simulink model "JX_Kinect20131119"  (Simulink 7.7)
settings: Solver=ode4  StartTime=0.0  StopTime=inf  FixedStep=sample_time  RelTol=1e-3
InitFcn:
  | sample_time=0.005;%0.004;%0.0025;%0.02;
  | DeltaT = 0.02;
  | g = 9.81;
  | H0 = g%0.3165;
  | Kl = 1;
  | 
  | Omega_r = 1.6;%for Horizontal reference
  | Zeta_r = 1; %for Horizontal reference
  | Omega = 1.8;%for Horizontal Control
  | Zeta = 0.5;    %for Horizontal Control
  | 
  | Omega_h_r = 2.5; %for vertical reference
  | Zeta_h_r = 0.8;  %for vertical reference
  | Omega_h = 2.7;    %for vertical control
  | Zeta_h = 0.8;         %for vertical control
  | PI=pi;
  | 
  | Mass = 1.15;
  | Acc_Max = 4;
  | Acc_Max_h = 4;
  | 
  | Max_RP = 60;
  | 
  | % for NN
  | n = 5;
  | r = 3;
  | n2 = 5;
  | NN_ST = 0.02;
  | 
  | GAMA_V = 6;
  | gama_V_e = 0.01;
  | 
  | GAMA_W = GAMA_V;
  | gama_W_e =0.01;
  | 
  | % deadzone
  | NN_Deadzone_Z = 0;
  | 
  | % inputs nomalizaton parameters
  | NN_Z_y_min = -3;
  | NN_Z_y_max = 0.5;
  | 
  | NN_Z_v_max = 8;
  | NN_Z_v_min = -NN_Z_v_max;
  | 
  | % alpha = 0.034;
  | alpha = 1;
  | % c_f = 0.0015;
  | c_f = 0.001;
  | c_y_tilt = 1*0.5;
  | 
  | %for WK paras
  | Heightcontrol = 0.08;
  | Scale_Factor=1;
  | yoffset=0;
  | 
  | load MaoBi_Oct04_2_int.mat
  | MB_Interp.time = [];
undefined symbols (not defined in the file or in its folder): DiscIntNeverNeededParam
libraries: simulink x7, dspadpt3 x3, nid_lib x2, X330_Control x2
(part 2 of 2)

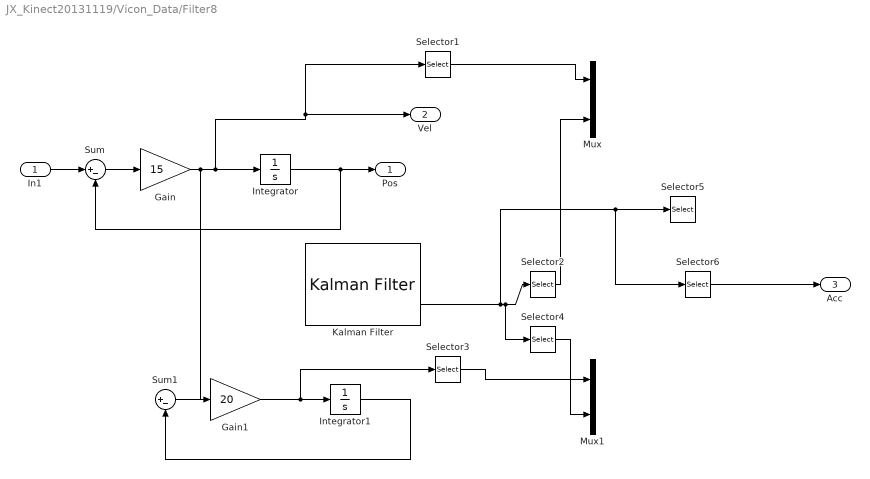
== system JX_Kinect20131119/Vicon_Data/Filter8 ==
  In1 : Inport
  Gain : Gain  Gain=15
  Gain1 : Gain  Gain=20
  Integrator : Integrator
  Integrator1 : Integrator
  Kalman Filter : dspadpt3/Kalman Filter  SystemSampleTime=-1  num_targets=1  sourceEnable=Always  isReset=on  X=zeros([9, 1])  P=zeros(9)  A=[1 sample_time sample_time*sample_time/2 zeros(1,6);0 1 sample_time zeros(1,6);0 0 1 zeros(1,6);0 0 0 1 sample_time sample_time*sample_time/2 0 0 0;zeros(1,4) 1 sample_time zeros(1,3);zeros(1,5) 1 zeros(1,3);zeros(1,6) 1 sample_time sample_time*sample_time/2;zeros(1,7) 1 sample_time;zeros(1,8) 1]  sourceMeasure=Specify via Dialog  H=[1 zeros(1,8); zeros(1,3) 1 zeros(1,5);zeros(1,6) 1 0 0]  Q=diag([0 0.001 0.001 0 0.001 0.001 0 0.001 0.001])  R=0.001*eye(3)  isOutputEstMeasure=on  isOutputEstState=on  isOutputEstError=off  isOutputPrdMeasure=off  isOutputPrdState=off  isOutputPrdError=off
  Mux : Mux  Inputs=2
  Mux1 : Mux  Inputs=2
  Selector1 : Selector  InputPortWidth=3  IndexOptions=Index vector (dialog)  Indices=[2]  OutputSizes=1
  Selector2 : Selector  InputPortWidth=9  IndexOptions=Index vector (dialog)  Indices=[5]  OutputSizes=1
  Selector3 : Selector  InputPortWidth=3  IndexOptions=Index vector (dialog)  Indices=[2]  OutputSizes=1
  Selector4 : Selector  InputPortWidth=9  IndexOptions=Index vector (dialog)  Indices=[6]  OutputSizes=1
  Selector5 : Selector  InputPortWidth=9  IndexOptions=Index vector (dialog)  Indices=[2 5 8]  OutputSizes=1
  Selector6 : Selector  InputPortWidth=9  IndexOptions=Index vector (dialog)  Indices=[3 6 9]  OutputSizes=1
  Sum : Sum  Inputs=|+-
  Sum1 : Sum  Inputs=|+-
  Pos : Outport
  Vel : Outport  Port=2
  Acc : Outport  Port=3
  wires:
  Selector6/1 -> Acc/1
  Selector4/1 -> Mux1/2
  Selector3/1 -> Mux1/1
  Selector2/1 -> Mux/2
  Integrator1/1 -> Sum1/2
  Gain1/1 -> Selector3/1, Integrator1/1
  Sum1/1 -> Gain1/1
  Kalman Filter/2 -> Selector6/1, Selector5/1, Selector2/1, Selector4/1
  Selector1/1 -> Mux/1
  In1/1 -> Sum/1
  Integrator/1 -> Sum/2, Pos/1
  Gain/1 -> Sum1/1, Vel/1, Selector1/1, Integrator/1
  Sum/1 -> Gain/1

== system JX_Kinect20131119/Vicon_Data/Raw Quad Pose from Vicon ==
  Constant : Constant
  Demux : Demux  Outputs=3
  Interpreted MATLAB Function : MATLABFcn  MATLABFcn=JXKinect05112013
  Process Vicon Raw Data1 : Subsystem
  Process Vicon Raw Data6 : Subsystem
  Process Vicon Raw Data7 : Subsystem
  Position_Vicon_JianXing : Outport
  Attitude_Vicon_JianXing : Outport  Port=2
  Position_Vicon_K platform : Outport  Port=3
  Attitude_Vicon_K platform : Outport  Port=4
  Position_Vicon_draw : Outport  Port=5
  Attitude_Vicon_draw : Outport  Port=6
  wires:
  Demux/3 -> Process Vicon Raw Data1/1(Vicon Raw)
  Process Vicon Raw Data1/1(Position) -> Position_Vicon_draw/1
  Process Vicon Raw Data1/2(Attitude) -> Attitude_Vicon_draw/1
  Demux/2 -> Process Vicon Raw Data7/1(Vicon Raw)
  Process Vicon Raw Data7/1(Position) -> Position_Vicon_K platform/1
  Process Vicon Raw Data7/2(Attitude) -> Attitude_Vicon_K platform/1
  Constant/1 -> Interpreted MATLAB Function/1
  Demux/1 -> Process Vicon Raw Data6/1(Vicon Raw)
  Process Vicon Raw Data6/1(Position) -> Position_Vicon_JianXing/1
  Process Vicon Raw Data6/2(Attitude) -> Attitude_Vicon_JianXing/1
  Interpreted MATLAB Function/1 -> Demux/1

== system JX_Kinect20131119/Kinect/Subsystem/Front or Center or Back ==
  Z: LH : Inport
  Z: LSh : Inport  Port=2
  Constant1 : Constant  Value=0
  Constant2 : Constant
  Constant3 : Constant  Value=-1
  If Back : Subsystem  TreatAsAtomicUnit=on
  If Center : Subsystem  TreatAsAtomicUnit=on
  If Front or Center or Back : If  IfExpression=u1 > 0.40  ElseIfExpressions=u1 >= 0.23
  If front : Subsystem  TreatAsAtomicUnit=on
  Merge3 : Merge  Inputs=3
  Subtract : Sum  Inputs=-+
  Y FrontCenterBack : Outport
  wires:
  Z: LH/1 -> Subtract/1
  Z: LSh/1 -> Subtract/2
  If Front or Center or Back/1 -> If front/Action
  If Front or Center or Back/2 -> If Center/Action
  If Front or Center or Back/3 -> If Back/Action
  If front/1(Out1) -> Merge3/1
  If Center/1(Out1) -> Merge3/2
  Constant2/1 -> If front/1(In1)
  Constant1/1 -> If Center/1(In1)
  Constant3/1 -> If Back/1(In1)
  If Back/1(Out1) -> Merge3/3
  Merge3/1 -> Y FrontCenterBack/1
  Subtract/1 -> If Front or Center or Back/1

== system JX_Kinect20131119/Kinect/Subsystem/Left or Center or Right ==
  X: LH : Inport
  X: LSh : Inport  Port=2
  Dead Zone : DeadZone  LowerValue=-0.14  UpperValue=0.14  SaturateOnIntegerOverflow=on
  Gain : Gain  Gain=2000
  Saturation : Saturate  UpperLimit=1  LowerLimit=-1
  Subtract : Sum  Inputs=+-
  X LeftCenterRight : Outport
  wires:
  X: LSh/1 -> Subtract/2
  X: LH/1 -> Subtract/1
  Subtract/1 -> Dead Zone/1
  Dead Zone/1 -> Gain/1
  Gain/1 -> Saturation/1
  Saturation/1 -> X LeftCenterRight/1

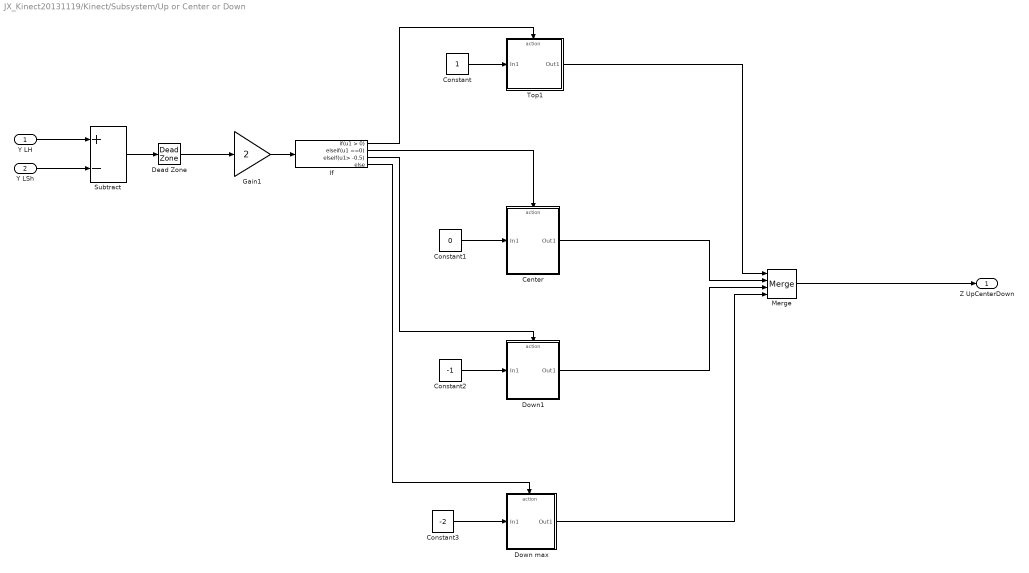
== system JX_Kinect20131119/Kinect/Subsystem/Up or Center or Down ==
  Y LH : Inport
  Y LSh : Inport  Port=2
  Center : Subsystem  TreatAsAtomicUnit=on
  Constant : Constant
  Constant1 : Constant  Value=0
  Constant2 : Constant  Value=-1
  Constant3 : Constant  Value=-2
  Dead Zone : DeadZone  LowerValue=-0.12  UpperValue=0.12  SaturateOnIntegerOverflow=on
  Down max : Subsystem  TreatAsAtomicUnit=on
  Down1 : Subsystem  TreatAsAtomicUnit=on
  Gain1 : Gain  Gain=2
  If : If  ElseIfExpressions=u1 ==0, u1> -0.5
  Merge : Merge  Inputs=4
  Subtract : Sum  Inputs=+-
  Top1 : Subsystem  TreatAsAtomicUnit=on
  Z UpCenterDown : Outport
  wires:
  Subtract/1 -> Dead Zone/1
  If/1 -> Top1/Action
  If/2 -> Center/Action
  If/3 -> Down1/Action
  If/4 -> Down max/Action
  Constant/1 -> Top1/1(In1)
  Dead Zone/1 -> Gain1/1
  Gain1/1 -> If/1
  Constant1/1 -> Center/1(In1)
  Constant2/1 -> Down1/1(In1)
  Constant3/1 -> Down max/1(In1)
  Center/1(Out1) -> Merge/2
  Down1/1(Out1) -> Merge/3
  Down max/1(Out1) -> Merge/4
  Top1/1(Out1) -> Merge/1
  Merge/1 -> Z UpCenterDown/1
  Y LH/1 -> Subtract/1
  Y LSh/1 -> Subtract/2

== system JX_Kinect20131119/Kinect/Subsystem1/Left or Center or Right ==
  X: RH : Inport
  X: RSh : Inport  Port=2
  Dead Zone : DeadZone  LowerValue=-0.12  UpperValue=0.12  SaturateOnIntegerOverflow=on
  Gain : Gain  Gain=2000
  Saturation : Saturate  UpperLimit=1  LowerLimit=-1
  Subtract : Sum  Inputs=+-
  LeftCenterRight : Outport
  wires:
  X: RSh/1 -> Subtract/2
  Subtract/1 -> Dead Zone/1
  Dead Zone/1 -> Gain/1
  Gain/1 -> Saturation/1
  Saturation/1 -> LeftCenterRight/1
  X: RH/1 -> Subtract/1

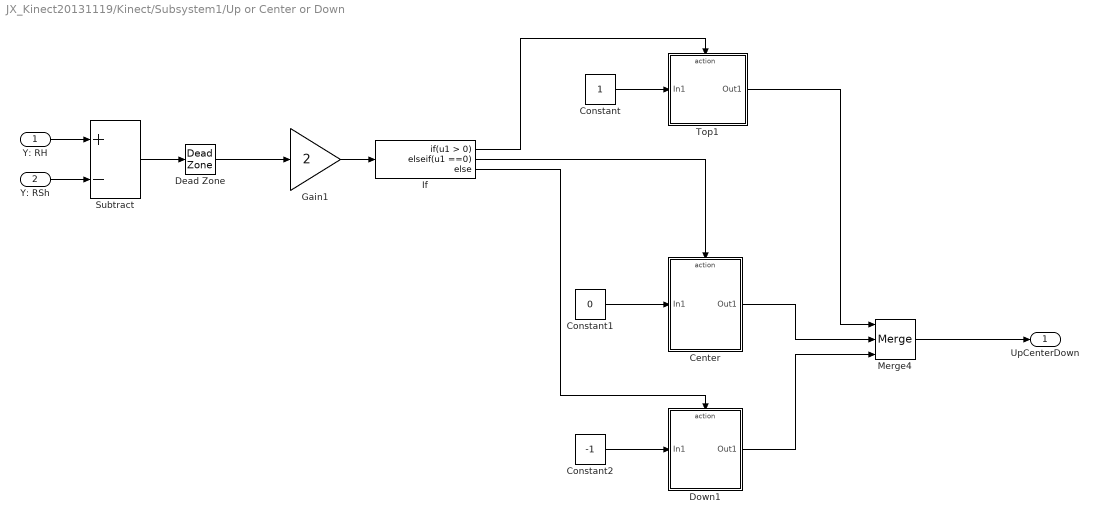
== system JX_Kinect20131119/Kinect/Subsystem1/Up or Center or Down ==
  Y: RH : Inport
  Y: RSh : Inport  Port=2
  Center : Subsystem  TreatAsAtomicUnit=on
  Constant : Constant
  Constant1 : Constant  Value=0
  Constant2 : Constant  Value=-1
  Dead Zone : DeadZone  LowerValue=-0.12  UpperValue=0.12  SaturateOnIntegerOverflow=on
  Down1 : Subsystem  TreatAsAtomicUnit=on
  Gain1 : Gain  Gain=2
  If : If  ElseIfExpressions=u1 ==0
  Merge4 : Merge  Inputs=3
  Subtract : Sum  Inputs=+-
  Top1 : Subsystem  TreatAsAtomicUnit=on
  UpCenterDown : Outport
  wires:
  Subtract/1 -> Dead Zone/1
  If/1 -> Top1/Action
  If/2 -> Center/Action
  Constant/1 -> Top1/1(In1)
  Dead Zone/1 -> Gain1/1
  Gain1/1 -> If/1
  Constant1/1 -> Center/1(In1)
  Constant2/1 -> Down1/1(In1)
  Center/1(Out1) -> Merge4/2
  Down1/1(Out1) -> Merge4/3
  Top1/1(Out1) -> Merge4/1
  Merge4/1 -> UpCenterDown/1
  Y: RH/1 -> Subtract/1
  Y: RSh/1 -> Subtract/2
  If/3 -> Down1/Action

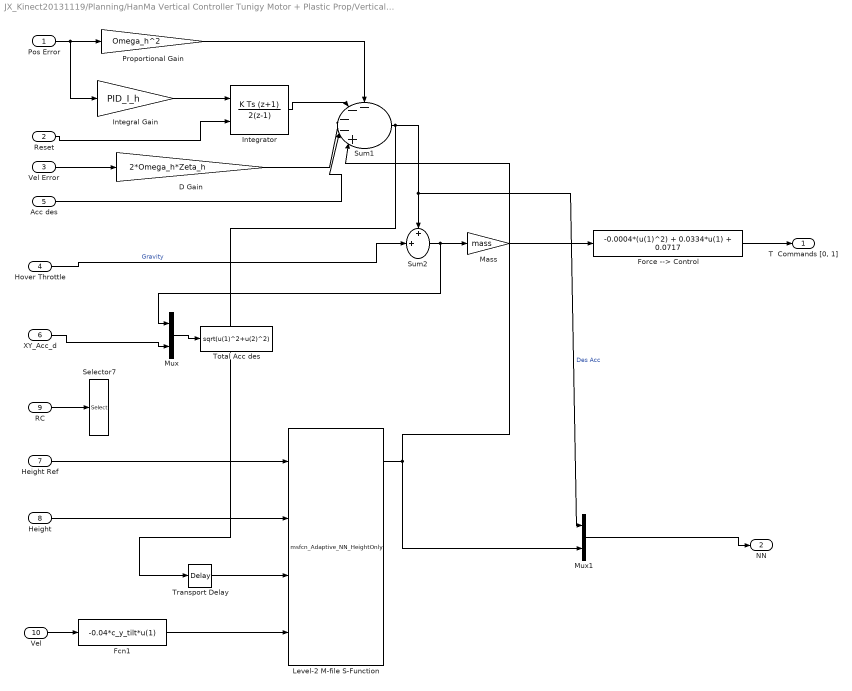
== system JX_Kinect20131119/Planning/HanMa Vertical Controller Tunigy Motor + Plastic Prop/Verticall Pos Controller ==
  Pos Error : Inport
  Reset : Inport  Port=2
  Vel Error : Inport  Port=3
  Hover Throttle : Inport  Port=4
  Acc des : Inport  Port=5
  XY_Acc_d : Inport  Port=6
  Height Ref : Inport  Port=7
  Height : Inport  Port=8
  RC : Inport  Port=9
  Vel : Inport  Port=10
  D Gain : Gain  Gain=2*Omega_h*Zeta_h  OutDataTypeStr=double
  Fcn1 : Fcn  Expr=-0.04*c_y_tilt*u(1)
  Force --> Control : Fcn  Expr=-0.0004*(u(1)^2) + 0.0334*u(1) + 0.0717
  Integral Gain : Gain  DisableCoverage=on  Gain=PID_I_h  ParamDataTypeStr=double  OutDataTypeStr=double
  Integrator : DiscreteIntegrator  DisableCoverage=on  IntegratorMethod=Integration: Trapezoidal  ExternalReset=rising  InitialConditionMode=State only (most efficient)  SampleTime=-1  OutDataTypeStr=double  UpperSaturationLimit=0.3  LowerSaturationLimit=-0.3  ICPrevOutput=DiscIntNeverNeededParam  ICPrevScaledInput=DiscIntNeverNeededParam
  Level-2 M-file S-Function : M-S-Function  FunctionName=msfcn_Adaptive_NN_HeightOnly  Parameters=n,r,n2,NN_ST,GAMA_V,gama_V_e,GAMA_W,gama_W_e,alpha,c_f,c_y_tilt,NN_Deadzone_Z,NN_Z_y_min,NN_Z_y_max,NN_Z_v_min,NN_Z_v_max
      mask Display: fprintf('Output Feedback NN \n Control Block')
  Mass : Gain  DisableCoverage=on  Gain=mass  ParamDataTypeStr=double  OutDataTypeStr=double
  Mux : Mux  Inputs=2
  Mux1 : Mux  Inputs=2
  Proportional Gain : Gain  DisableCoverage=on  Gain=Omega_h^2  ParamDataTypeStr=double  OutDataTypeStr=double
  Selector7 : Selector  InputPortWidth=8  IndexOptions=Index vector (dialog)  Indices=[6]  OutputSizes=1
  Sum1 : Sum  DisableCoverage=on  Inputs=----+|  AccumDataTypeStr=double  OutDataTypeStr=double  SampleTime=0.02
  Sum2 : Sum  DisableCoverage=on  Inputs=++|  AccumDataTypeStr=double  OutDataTypeStr=double  SampleTime=0.02
  Total Acc des : Fcn  Expr=sqrt(u(1)^2+u(2)^2)
  Transport Delay : TransportDelay  DelayTime=0.02
  "T  Commands [0, 1]" : Outport
  NN : Outport  Port=2
  wires:
  Force --> Control/1 -> "T  Commands [0, 1]"/1
  Sum2/1 -> Mux/1, Mass/1
  XY_Acc_d/1 -> Mux/2
  Mux/1 -> Total Acc des/1
  Mass/1 -> Force --> Control/1
  Sum1/1 -> Transport Delay/1, Sum2/1, Mux1/1  "Des Acc"
  Hover Throttle/1 -> Sum2/2  "Gravity"
  Acc des/1 -> Sum1/4
  D Gain/1 -> Sum1/3
  Vel Error/1 -> D Gain/1
  Reset/1 -> Integrator/2
  Pos Error/1 -> Integral Gain/1, Proportional Gain/1
  Proportional Gain/1 -> Sum1/1
  Integrator/1 -> Sum1/2
  Integral Gain/1 -> Integrator/1
  Height Ref/1 -> Level-2 M-file S-Function/1
  Level-2 M-file S-Function/1 -> Mux1/2, Sum1/5
  RC/1 -> Selector7/1
  Fcn1/1 -> Level-2 M-file S-Function/4
  Transport Delay/1 -> Level-2 M-file S-Function/3
  Mux1/1 -> NN/1
  Vel/1 -> Fcn1/1
  Height/1 -> Level-2 M-file S-Function/2

== system JX_Kinect20131119/Planning/Yaw Controller/Heading ==
  u : Inport  SampleTime=SampleTime
  RESET : Inport  Port=2  SampleTime=SampleTime
  Integral Gain : Gain  DisableCoverage=on  Gain=I  ParamMin=IParamMin  ParamMax=IParamMax  ParamDataTypeStr=IParamDataTypeStr  OutMin=IOutMin  OutMax=IOutMax  OutDataTypeStr=IOutDataTypeStr
  Integrator : DiscreteIntegrator  DisableCoverage=on  IntegratorMethod=Integration: Trapezoidal  ExternalReset=rising  InitialCondition=InitialConditionForIntegrator  InitialConditionMode=State only (most efficient)  SampleTime=-1  OutMin=IntegratorOutMin  OutMax=IntegratorOutMax  OutDataTypeStr=IntegratorOutDataTypeStr  ICPrevOutput=DiscIntNeverNeededParam  ICPrevScaledInput=DiscIntNeverNeededParam
  Proportional Gain : Gain  DisableCoverage=on  Gain=P  ParamMin=PParamMin  ParamMax=PParamMax  ParamDataTypeStr=PParamDataTypeStr  OutMin=POutMin  OutMax=POutMax  OutDataTypeStr=POutDataTypeStr
  Saturation : Saturate  UpperLimit=UpperSaturationLimit  LowerLimit=LowerSaturationLimit  LinearizeAsGain=off  OutMin=SaturationOutMin  OutMax=SaturationOutMax  OutDataTypeStr=SaturationOutDataTypeStr
  Sum : Sum  DisableCoverage=on  Inputs=++|  AccumDataTypeStr=SumAccumDataTypeStr  OutMin=SumOutMin  OutMax=SumOutMax  OutDataTypeStr=SumOutDataTypeStr
  y : Outport  InitialOutput=0
  wires:
  Sum/1 -> Saturation/1
  Saturation/1 -> y/1
  RESET/1 -> Integrator/2
  Proportional Gain/1 -> Sum/1
  Integrator/1 -> Sum/2
  Integral Gain/1 -> Integrator/1
  u/1 -> Proportional Gain/1, Integral Gain/1

== system JX_Kinect20131119/Vicon_Data/Raw Quad Pose from Vicon/Process Vicon Raw Data1 ==
  note: Z
  note: Y
  note: X
  Vicon Raw : Inport
  Add1 : Sum  Inputs=-+
  Constant1 : Constant  Value=pi  OutDataTypeStr=double
  Demux : Demux  Outputs=6
  Flip_pi1 : Subsystem
      mask Type: Flip -pi to pi
      mask Description: Flips the inputs into the range -pi to pi
      mask Help: Flips the inputs into the range -pi to pi
      mask Display: disp('Flip_pi')
  Gain1 : Gain  Gain=0.001
  Gain3 : Gain  Gain=-1
  Gain6 : Gain  Gain=-0.001
  Gain7 : Gain  Gain=-0.001
  Matrix Concatenate1 : Concatenate  NumInputs=3  Mode=Multidimensional array
  Matrix Concatenate13 : Concatenate  NumInputs=3  Mode=Multidimensional array
  Position : Outport
  Attitude : Outport  Port=2
  wires:
  Matrix Concatenate1/1 -> Attitude/1
  Vicon Raw/1 -> Demux/1
  Matrix Concatenate13/1 -> Position/1
  Flip_pi1/1(Angle_Flip) -> Matrix Concatenate1/1
  Demux/5 -> Matrix Concatenate1/2  "pitch"
  Gain3/1 -> Flip_pi1/1(Angle)
  Add1/1 -> Gain3/1
  Gain7/1 -> Matrix Concatenate13/3
  Gain6/1 -> Matrix Concatenate13/2
  Demux/4 -> Add1/1  "roll"
  Demux/3 -> Gain7/1
  Demux/2 -> Gain6/1
  Demux/1 -> Gain1/1
  Gain1/1 -> Matrix Concatenate13/1
  Demux/6 -> Matrix Concatenate1/3  "yaw"
  Constant1/1 -> Add1/2

== system JX_Kinect20131119/Vicon_Data/Raw Quad Pose from Vicon/Process Vicon Raw Data6 ==
  note: Z
  note: Y
  note: X
  Vicon Raw : Inport
  Add1 : Sum  Inputs=-+
  Constant1 : Constant  Value=pi  OutDataTypeStr=double
  Demux : Demux  Outputs=6
  Flip_pi1 : Subsystem
      mask Type: Flip -pi to pi
      mask Description: Flips the inputs into the range -pi to pi
      mask Help: Flips the inputs into the range -pi to pi
      mask Display: disp('Flip_pi')
  Gain1 : Gain  Gain=0.001
  Gain3 : Gain  Gain=-1
  Gain6 : Gain  Gain=-0.001
  Gain7 : Gain  Gain=-0.001
  Matrix Concatenate1 : Concatenate  NumInputs=3  Mode=Multidimensional array
  Matrix Concatenate13 : Concatenate  NumInputs=3  Mode=Multidimensional array
  Position : Outport
  Attitude : Outport  Port=2
  wires:
  Matrix Concatenate1/1 -> Attitude/1
  Vicon Raw/1 -> Demux/1
  Matrix Concatenate13/1 -> Position/1
  Flip_pi1/1(Angle_Flip) -> Matrix Concatenate1/1
  Demux/5 -> Matrix Concatenate1/2  "pitch"
  Gain3/1 -> Flip_pi1/1(Angle)
  Add1/1 -> Gain3/1
  Gain7/1 -> Matrix Concatenate13/3
  Gain6/1 -> Matrix Concatenate13/2
  Demux/4 -> Add1/1  "roll"
  Demux/3 -> Gain7/1
  Demux/2 -> Gain6/1
  Demux/1 -> Gain1/1
  Gain1/1 -> Matrix Concatenate13/1
  Demux/6 -> Matrix Concatenate1/3  "yaw"
  Constant1/1 -> Add1/2

== system JX_Kinect20131119/Vicon_Data/Raw Quad Pose from Vicon/Process Vicon Raw Data7 ==
  note: X
  note: Y
  note: Z
  Vicon Raw : Inport
  Add1 : Sum  Inputs=-+
  Constant1 : Constant  Value=pi  OutDataTypeStr=double
  Demux : Demux  Outputs=6
  Flip_pi1 : Subsystem
      mask Type: Flip -pi to pi
      mask Description: Flips the inputs into the range -pi to pi
      mask Help: Flips the inputs into the range -pi to pi
      mask Display: disp('Flip_pi')
  Gain1 : Gain  Gain=0.001
  Gain3 : Gain  Gain=-1
  Gain6 : Gain  Gain=-0.001
  Gain7 : Gain  Gain=-0.001
  Matrix Concatenate1 : Concatenate  NumInputs=3  Mode=Multidimensional array
  Matrix Concatenate13 : Concatenate  NumInputs=3  Mode=Multidimensional array
  Position : Outport
  Attitude : Outport  Port=2
  wires:
  Constant1/1 -> Add1/2
  Demux/6 -> Matrix Concatenate1/3  "yaw"
  Gain1/1 -> Matrix Concatenate13/1
  Demux/1 -> Gain1/1
  Demux/2 -> Gain6/1
  Demux/3 -> Gain7/1
  Demux/4 -> Add1/1  "roll"
  Gain6/1 -> Matrix Concatenate13/2
  Gain7/1 -> Matrix Concatenate13/3
  Add1/1 -> Gain3/1
  Gain3/1 -> Flip_pi1/1(Angle)
  Demux/5 -> Matrix Concatenate1/2  "pitch"
  Flip_pi1/1(Angle_Flip) -> Matrix Concatenate1/1
  Matrix Concatenate13/1 -> Position/1
  Vicon Raw/1 -> Demux/1
  Matrix Concatenate1/1 -> Attitude/1

== system JX_Kinect20131119/Kinect/Subsystem/Front or Center or Back/If Back ==
  In1 : Inport
  Action Port : ActionPort  ActionType=else
  Out1 : Outport
  wires:
  In1/1 -> Out1/1

== system JX_Kinect20131119/Kinect/Subsystem/Front or Center or Back/If Center ==
  In1 : Inport
  Action Port : ActionPort  ActionType=elseif
  Out1 : Outport
  wires:
  In1/1 -> Out1/1

== system JX_Kinect20131119/Kinect/Subsystem/Front or Center or Back/If front ==
  In1 : Inport
  Action Port : ActionPort  ActionType=then
  Out1 : Outport
  wires:
  In1/1 -> Out1/1

== system JX_Kinect20131119/Kinect/Subsystem/Up or Center or Down/Center ==
  In1 : Inport
  Action Port : ActionPort  ActionType=elseif
  Out1 : Outport
  wires:
  In1/1 -> Out1/1

== system JX_Kinect20131119/Kinect/Subsystem/Up or Center or Down/Down max ==
  In1 : Inport
  Action Port : ActionPort  ActionType=else
  Out1 : Outport
  wires:
  In1/1 -> Out1/1

== system JX_Kinect20131119/Kinect/Subsystem/Up or Center or Down/Down1 ==
  In1 : Inport
  Action Port : ActionPort  ActionType=elseif
  Out1 : Outport
  wires:
  In1/1 -> Out1/1

== system JX_Kinect20131119/Kinect/Subsystem/Up or Center or Down/Top1 ==
  In1 : Inport
  Action Port : ActionPort  ActionType=then
  Out1 : Outport
  wires:
  In1/1 -> Out1/1

== system JX_Kinect20131119/Kinect/Subsystem1/Up or Center or Down/Center ==
  In1 : Inport
  Action Port : ActionPort  ActionType=elseif
  Out1 : Outport
  wires:
  In1/1 -> Out1/1

== system JX_Kinect20131119/Kinect/Subsystem1/Up or Center or Down/Down1 ==
  In1 : Inport
  Action Port : ActionPort  ActionType=else
  Out1 : Outport
  wires:
  In1/1 -> Out1/1

== system JX_Kinect20131119/Kinect/Subsystem1/Up or Center or Down/Top1 ==
  In1 : Inport
  Action Port : ActionPort  ActionType=then
  Out1 : Outport
  wires:
  In1/1 -> Out1/1

== system JX_Kinect20131119/Vicon_Data/Raw Quad Pose from Vicon/Process Vicon Raw Data1/Flip_pi1 ==
  Angle : Inport
  Add : Sum  Inputs=-+
  Compare To Constant1 : simulink/Logic and Bit Operations/Compare To Constant  SystemSampleTime=-1  relop=>  const=pi  LogicOutDataTypeMode=uint8  ZeroCross=off
  Constant : Constant  Value=2*pi
  Data Type Duplicate : DataTypeDuplicate
  Flip_0_to_2pi : Subsystem
      mask Type: Flip zero to 2pi
      mask Description: Flips the inputs into the range zero to +2pi
      mask Help: Flips the inputs into the range zero to +2pi
      mask Display: disp('Flip_0_2pi')
  Switch : Switch  Criteria=u2 ~= 0
  Angle_Flip : Outport
  wires:
  Angle/1 -> Flip_0_to_2pi/1(Angle), Data Type Duplicate/2
  Flip_0_to_2pi/1(Angle_Flip) -> Switch/3, Compare To Constant1/1, Add/2
  Compare To Constant1/1 -> Switch/2
  Constant/1 -> Add/1
  Add/1 -> Switch/1
  Switch/1 -> Angle_Flip/1, Data Type Duplicate/1

== system JX_Kinect20131119/Vicon_Data/Raw Quad Pose from Vicon/Process Vicon Raw Data6/Flip_pi1 ==
  Angle : Inport
  Add : Sum  Inputs=-+
  Compare To Constant1 : simulink/Logic and Bit Operations/Compare To Constant  SystemSampleTime=-1  relop=>  const=pi  LogicOutDataTypeMode=uint8  ZeroCross=off
  Constant : Constant  Value=2*pi
  Data Type Duplicate : DataTypeDuplicate
  Flip_0_to_2pi : Subsystem
      mask Type: Flip zero to 2pi
      mask Description: Flips the inputs into the range zero to +2pi
      mask Help: Flips the inputs into the range zero to +2pi
      mask Display: disp('Flip_0_2pi')
  Switch : Switch  Criteria=u2 ~= 0
  Angle_Flip : Outport
  wires:
  Angle/1 -> Flip_0_to_2pi/1(Angle), Data Type Duplicate/2
  Flip_0_to_2pi/1(Angle_Flip) -> Switch/3, Compare To Constant1/1, Add/2
  Compare To Constant1/1 -> Switch/2
  Constant/1 -> Add/1
  Add/1 -> Switch/1
  Switch/1 -> Angle_Flip/1, Data Type Duplicate/1

== system JX_Kinect20131119/Vicon_Data/Raw Quad Pose from Vicon/Process Vicon Raw Data7/Flip_pi1 ==
  Angle : Inport
  Add : Sum  Inputs=-+
  Compare To Constant1 : simulink/Logic and Bit Operations/Compare To Constant  SystemSampleTime=-1  relop=>  const=pi  LogicOutDataTypeMode=uint8  ZeroCross=off
  Constant : Constant  Value=2*pi
  Data Type Duplicate : DataTypeDuplicate
  Flip_0_to_2pi : Subsystem
      mask Type: Flip zero to 2pi
      mask Description: Flips the inputs into the range zero to +2pi
      mask Help: Flips the inputs into the range zero to +2pi
      mask Display: disp('Flip_0_2pi')
  Switch : Switch  Criteria=u2 ~= 0
  Angle_Flip : Outport
  wires:
  Switch/1 -> Data Type Duplicate/1, Angle_Flip/1
  Add/1 -> Switch/1
  Constant/1 -> Add/1
  Compare To Constant1/1 -> Switch/2
  Flip_0_to_2pi/1(Angle_Flip) -> Add/2, Compare To Constant1/1, Switch/3
  Angle/1 -> Data Type Duplicate/2, Flip_0_to_2pi/1(Angle)

== system JX_Kinect20131119/Vicon_Data/Raw Quad Pose from Vicon/Process Vicon Raw Data1/Flip_pi1/Flip_0_to_2pi ==
  Angle : Inport
  Add : Sum
  Compare To Constant1 : simulink/Logic and Bit Operations/Compare To Constant  SystemSampleTime=-1  relop=<  const=0  LogicOutDataTypeMode=uint8  ZeroCross=off
  Constant : Constant  Value=2*pi
  Data Type Duplicate : DataTypeDuplicate
  Flip_2pi : Subsystem
      mask Type: Flip -2pi to 2pi
      mask Description: Flips the inputs into the range -2pi to +2pi
      mask Help: Flips the inputs into the range -2pi to +2pi
      mask Display: disp('Flip_2pi')
  Switch : Switch  Criteria=u2 ~= 0
  Angle_Flip : Outport
  wires:
  Flip_2pi/1(Angle_Flip) -> Compare To Constant1/1, Add/2, Switch/3
  Compare To Constant1/1 -> Switch/2
  Constant/1 -> Add/1
  Add/1 -> Switch/1
  Angle/1 -> Flip_2pi/1(Angle), Data Type Duplicate/2
  Switch/1 -> Angle_Flip/1, Data Type Duplicate/1

== system JX_Kinect20131119/Vicon_Data/Raw Quad Pose from Vicon/Process Vicon Raw Data6/Flip_pi1/Flip_0_to_2pi ==
  Angle : Inport
  Add : Sum
  Compare To Constant1 : simulink/Logic and Bit Operations/Compare To Constant  SystemSampleTime=-1  relop=<  const=0  LogicOutDataTypeMode=uint8  ZeroCross=off
  Constant : Constant  Value=2*pi
  Data Type Duplicate : DataTypeDuplicate
  Flip_2pi : Subsystem
      mask Type: Flip -2pi to 2pi
      mask Description: Flips the inputs into the range -2pi to +2pi
      mask Help: Flips the inputs into the range -2pi to +2pi
      mask Display: disp('Flip_2pi')
  Switch : Switch  Criteria=u2 ~= 0
  Angle_Flip : Outport
  wires:
  Flip_2pi/1(Angle_Flip) -> Compare To Constant1/1, Add/2, Switch/3
  Compare To Constant1/1 -> Switch/2
  Constant/1 -> Add/1
  Add/1 -> Switch/1
  Angle/1 -> Flip_2pi/1(Angle), Data Type Duplicate/2
  Switch/1 -> Angle_Flip/1, Data Type Duplicate/1

== system JX_Kinect20131119/Vicon_Data/Raw Quad Pose from Vicon/Process Vicon Raw Data7/Flip_pi1/Flip_0_to_2pi ==
  Angle : Inport
  Add : Sum
  Compare To Constant1 : simulink/Logic and Bit Operations/Compare To Constant  SystemSampleTime=-1  relop=<  const=0  LogicOutDataTypeMode=uint8  ZeroCross=off
  Constant : Constant  Value=2*pi
  Data Type Duplicate : DataTypeDuplicate
  Flip_2pi : Subsystem
      mask Type: Flip -2pi to 2pi
      mask Description: Flips the inputs into the range -2pi to +2pi
      mask Help: Flips the inputs into the range -2pi to +2pi
      mask Display: disp('Flip_2pi')
  Switch : Switch  Criteria=u2 ~= 0
  Angle_Flip : Outport
  wires:
  Switch/1 -> Data Type Duplicate/1, Angle_Flip/1
  Angle/1 -> Data Type Duplicate/2, Flip_2pi/1(Angle)
  Add/1 -> Switch/1
  Constant/1 -> Add/1
  Compare To Constant1/1 -> Switch/2
  Flip_2pi/1(Angle_Flip) -> Switch/3, Add/2, Compare To Constant1/1

== system JX_Kinect20131119/Vicon_Data/Raw Quad Pose from Vicon/Process Vicon Raw Data1/Flip_pi1/Flip_0_to_2pi/Flip_2pi ==
  Angle : Inport
  Bias : Bias  Bias=-2*pi
  Constant : Constant  Value=2*pi
  Data Type Duplicate : DataTypeDuplicate
  Modulo : Math  Operator=mod  SaturateOnIntegerOverflow=on
  Sign1 : Signum
  Switch : Switch
  Angle_Flip : Outport
  wires:
  Angle/1 -> Modulo/1, Sign1/1, Data Type Duplicate/1
  Constant/1 -> Modulo/2
  Modulo/1 -> Bias/1, Switch/1
  Sign1/1 -> Switch/2
  Bias/1 -> Switch/3
  Switch/1 -> Angle_Flip/1, Data Type Duplicate/2

== system JX_Kinect20131119/Vicon_Data/Raw Quad Pose from Vicon/Process Vicon Raw Data6/Flip_pi1/Flip_0_to_2pi/Flip_2pi ==
  Angle : Inport
  Bias : Bias  Bias=-2*pi
  Constant : Constant  Value=2*pi
  Data Type Duplicate : DataTypeDuplicate
  Modulo : Math  Operator=mod  SaturateOnIntegerOverflow=on
  Sign1 : Signum
  Switch : Switch
  Angle_Flip : Outport
  wires:
  Angle/1 -> Modulo/1, Sign1/1, Data Type Duplicate/1
  Constant/1 -> Modulo/2
  Modulo/1 -> Bias/1, Switch/1
  Sign1/1 -> Switch/2
  Bias/1 -> Switch/3
  Switch/1 -> Angle_Flip/1, Data Type Duplicate/2

== system JX_Kinect20131119/Vicon_Data/Raw Quad Pose from Vicon/Process Vicon Raw Data7/Flip_pi1/Flip_0_to_2pi/Flip_2pi ==
  Angle : Inport
  Bias : Bias  Bias=-2*pi
  Constant : Constant  Value=2*pi
  Data Type Duplicate : DataTypeDuplicate
  Modulo : Math  Operator=mod  SaturateOnIntegerOverflow=on
  Sign1 : Signum
  Switch : Switch
  Angle_Flip : Outport
  wires:
  Switch/1 -> Data Type Duplicate/2, Angle_Flip/1
  Bias/1 -> Switch/3
  Sign1/1 -> Switch/2
  Modulo/1 -> Switch/1, Bias/1
  Constant/1 -> Modulo/2
  Angle/1 -> Data Type Duplicate/1, Sign1/1, Modulo/1

== matlab function Planning/Yaw Controller/MATLAB Function ==
  data: u input double; y output double
function y = fcn(u)
%#codegen
y = u;
if y > pi    
    y = y - 2*pi;
elseif y < -pi
        y = y + 2*pi;
end

== stateflow chart Planning/Trajectory Logic/UAV SF ==
  state Landing
    state Descending
      en:PosDesired = Pos;
      du:PosDesired[2] = (0.1- PosDesired[2])*1*DeltaT + PosDesired[2] ;
    state CutThrottle
      en: PWM=1600;
      du:HoverThrottle = (0.0- HoverThrottle)*3*DeltaT + HoverThrottle ;
    (default) -> Descending
    Descending -> CutThrottle : [Pos[2] >(0.0 -0.1)]
  state AirBorne
    state TakeOff
      du:HoverThrottle = (H0 - HoverThrottle)*3*DeltaT + HoverThrottle ;
    state Kinect
      state Initialise
        en:
        PosDesired[0]=0, PosDesired[1]=-0,PosDesired[2]= -1.5,PosDesired[3]=0;
        LeftRight = 0;
        UpDown = 0;
        FrontBack = 0;
        Toggle = 1;
        ClawStatus = 1;
        Rotation = 0;
        PWM = 1690;
        LXC=0; LYC=0; LZC=0; RXYC=0; safechecker = 2;
      state Hover
        en:
        PosDesired[0]=0+LeftRight, PosDesired[1]=0+FrontBack,PosDesired[2]= -1.5+UpDown,PosDesired[3] = 0+Rotation;
        LHRH = 0;
        XYZchecker=0;
      state KinectTrack
        state CheckLEFTZ
          state ZCenter
            en:
            UpDown=UpDown+0;
            LZC=0;
            LHRH = 3;
          state ZDown
            en:
            UpDown=UpDown+0.02;
            LHRH = 3;
          state ZUp
            en:
            UpDown=UpDown-0.02;
            LHRH = 3;
          (junction 64) -> ZUp [order 3] : [LeftHand[2]==1]
          (junction 64) -> ZDown [order 1] : [LeftHand[2]== -1]
          (junction 64) -> ZCenter [order 2] : [LeftHand[2]==0]
          (default) -> (junction 64)
        state CheckLEFTX
          state XLeft
            en:
            LeftRight=LeftRight-0.02;
            LHRH=1;
          state XRight
            en:
            LeftRight=LeftRight+0.02;
            LHRH=1;
          state XCenter
            en:
            LeftRight=LeftRight+0;
            LXC=0;
            LHRH=1;
          (junction 62) -> XRight [order 1] : [LeftHand[0]== -1]
          (default) -> (junction 62)
          (junction 62) -> XLeft [order 3] : [LeftHand[0]==1]
          (junction 62) -> XCenter [order 2] : [LeftHand[0]==0]
        state CheckRIGHTXY
          state ToggleOpen
            en:
            ClawStatus=1;
            Toggle=2;
            LHRH=4;
          state ToggleClose
            en:
            ClawStatus=0;
            Toggle=2;
            LHRH=4;
          state RightHanddown
            en:
            Toggle=1;
            LHRH = 4;
          state ContinuousHandUp
            en:
            LHRH=4;
          state Heading
            state Clockwise
              en:
              Rotation=Rotation+0.01;
              Toggle=1;
              LHRH=4;
            state Neutral
              en:
              Rotation = Rotation +0;
              RXYC=0;
              Toggle=1;
              LHRH = 4;
            state AntiClockwise
              en:
              Rotation = Rotation - 0.01;
              Toggle=1;
              LHRH = 4;
            (default) -> (junction 72)
            (junction 72) -> Clockwise [order 3] : [RightHand[1]==1]
            (junction 72) -> AntiClockwise [order 1] : [RightHand[1]==-1]
            (junction 72) -> Neutral [order 2] : [RightHand[1]==0]
          (default) -> (junction 70)
          (junction 70) -> (junction 77) [order 3] : [RightHand[0]==1]
          (junction 70) -> RightHanddown [order 2] : [RightHand[0]== -1]
          (junction 70) -> Heading [order 1] : [RightHand[0]==0]
          (junction 77) -> ContinuousHandUp [order 1] : [Toggle==2]
          (junction 76) -> ToggleClose [order 1] : [ClawStatus==1]
          (junction 77) -> (junction 76) [order 2] : [Toggle==1]
          (junction 76) -> ToggleOpen [order 2] : [ClawStatus==0]
        state CLAW
          state OpenMax
            en:
            PWM = 1690;
            LHRH = 5;
          state CloseMax
            en:
            PWM = 1200;
            LHRH = 5;
          state OpenClaw
            en:
            PWM = PWM+100;
            LHRH = 5;
          state CloseClaw
            en:
            PWM = PWM-100;
            LHRH = 5;
          (junction 74) -> (junction 71) [order 1] : [ClawStatus==0]
          (junction 74) -> (junction 73) [order 2] : [ClawStatus==1]
          (junction 73) -> OpenMax [order 1] : [PWM>=1680]
          (junction 73) -> OpenClaw [order 2] : [PWM<1680]
          (junction 71) -> CloseClaw [order 2] : [PWM>1180]
          (junction 71) -> CloseMax [order 1] : [PWM<=1180]
          (default) -> (junction 74)
        state CheckLEFTY
          state YCenter
            en:
            FrontBack=FrontBack+0;
            LYC=0;
            LHRH = 2;
          state YFront
            en:
            FrontBack=FrontBack-0.02;
            LHRH = 2;
          state YBack
            en:
            FrontBack=FrontBack+0.02;
            LHRH = 2;
          (default) -> (junction 63)
          (junction 63) -> YFront [order 3] : [LeftHand[1]==1]
          (junction 63) -> YCenter [order 2] : [LeftHand[1]==0]
          (junction 63) -> YBack [order 1] : [LeftHand[1]== -1]
        CheckLEFTX -> CheckLEFTY : [(LHRH==1)]
        CheckLEFTY -> CheckLEFTZ : [(LHRH==2)]
        (junction 68) -> CheckLEFTX [order 2] : [LeftHand[2]~= -2]
        CheckLEFTZ -> CheckRIGHTXY : [(LHRH==3)]
        (junction 68) -> CheckRIGHTXY [order 1] : [LeftHand[2]== -2]
        CheckRIGHTXY -> CLAW : [LHRH ==4]
        (default) -> (junction 68)
      state Constraint
        state PositionConstraint
          state Xpositive
            en:
            LeftRight=2;
          state Xnegative
            en:
            LeftRight=-2;
          state Ypositive
            en:
            FrontBack=2;
          state Ynegative
            en:
            FrontBack=-2;
          state Zpositive
            en:
            UpDown=0.77;
          state Znegative
            en:
            UpDown=-1;
          state RotateACW
            en:
            Rotation=-3.1;
          state RotateCW
            en:
            Rotation=3.1;
          state Contained
            en:
            LHRH = 7;
          (junction 65) -> Contained [order 1] : [Rotation>=-3.1]
          Znegative -> (junction 75)
          (default) -> (junction 67)
          (junction 67) -> Xpositive [order 2] : [LeftRight>2]
          (junction 66) -> Xnegative [order 2] : [LeftRight<-2]
          (junction 80) -> Ypositive [order 2] : [FrontBack>2]
          (junction 79) -> Ynegative [order 2] : [FrontBack<-2]
          (junction 78) -> Zpositive [order 2] : [UpDown>0.77]
          Xnegative -> (junction 80)
          (junction 78) -> (junction 69) [order 1] : [UpDown<=0.77]
          Ypositive -> (junction 79)
          (junction 79) -> (junction 78) [order 1] : [FrontBack>=-2]
          (junction 69) -> (junction 75) [order 1] : [UpDown>=-1]
          RotateACW -> Contained
          RotateCW -> (junction 65)
          (junction 65) -> RotateACW [order 2] : [Rotation<-3.1]
          (junction 75) -> (junction 65) [order 1] : [Rotation<=3.1]
          (junction 75) -> RotateCW [order 2] : [Rotation>3.1]
          Ynegative -> (junction 78)
          Zpositive -> (junction 69)
          (junction 69) -> Znegative [order 2] : [UpDown<-1]
          (junction 67) -> (junction 66) [order 1] : [LeftRight<=2]
          Xpositive -> (junction 66)
          (junction 66) -> (junction 80) [order 1] : [LeftRight>=-2]
          (junction 80) -> (junction 79) [order 1] : [FrontBack<=2]
        state ALLGreen
          en:
          LHRH = 7;
        (junction 81) -> PositionConstraint [order 2] : [(LeftRight > 2)|(LeftRight<-2)|(FrontBack>2)|(FrontBack<-2)|(UpDown>0.77)|(UpDown<-1)|(Rotation>3.1)|(Rotation<-3.1)]
        (junction 81) -> ALLGreen [order 1] : [(LeftRight<=2)&(LeftRight>=-2)&(FrontBack<=2)&(FrontBack>=-2)&(UpDown<=0.77)&(UpDown>=-1)&(Rotation<=3.1)&(Rotation>=-3.1)]
        PositionConstraint -> ALLGreen : [(LeftRight<=2)&(LeftRight>=-2)&(FrontBack<=2)&(FrontBack>=-2)&(UpDown<=0.77)&(UpDown>=-1)&(Rotation<=3.1)&(Rotation>=-3.1)]
        (default) -> (junction 81)
      KinectTrack -> Hover [order 1] : [KinectTracking==0]
      Hover -> KinectTrack : [KinectTracking==1]
      KinectTrack -> Constraint [order 2] : [(LHRH==5)]
      (default) -> Initialise
      Initialise -> Hover : after (3,sec)
      Constraint -> Hover : [LHRH==7]
    state Safety
      state Descent1
        descentrate=descentrate+0.02;
      state Descent
        en:PosDesired[0] = PerchPos[0]; PosDesired[1] = PerchPos[1];PosDesired[2] = PerchPos[2]-0.50+descentrate;
      state Prelanding
        en:PosDesired[0] = PerchPos[0]; PosDesired[1] = PerchPos[1];PosDesired[2] = PerchPos[2]-0.8 ;
        descentrate=0;
      state SafyHover
        en:PosDesired = Pos; PosDesired[2]= -1.5;
      (default) -> SafyHover
      Descent1 -> Descent : after (0.5,sec)
      Descent -> Descent1 [order 2] : [PerchError < 0.02]
      Descent -> Prelanding [order 1] : after (5,sec)
      Prelanding -> Descent : [PerchError < 0.01]
      SafyHover -> Prelanding : after (3, sec)
    (default) -> TakeOff : {PosDesired = Pos;  PosDesired[2] =-1.2;}
    TakeOff -> Kinect [order 1] : after (7,sec)
    TakeOff -> Safety [order 2] : [RC[5] > 0.5]
    Kinect -> Safety : [RC[5] > 0.5]
  (default) -> Landing : {HoverThrottle = 0;}
  AirBorne -> Landing : [RC[6] < -0.5]
  Landing -> AirBorne : [RC[6] > 0.5]
  data: PosDesired output double size=4; HoverThrottle output double size=1; Mode output uint8 size=1; RC input double size=8; Pos input double size=4; PerchPos input double size=4; DeltaT parameter double size=1; H0 parameter double size=1; Kl parameter double size=1; VelCmd local double size=2 =0; PWM output double; PerchError input double; PI parameter double size=1; draw input double size=3; descentrate local double; LeftHand input double; KinectTracking input double; UpDown local double; FrontBack local double; XYZchecker local double; RightHand input double; ClawStatus local double; LHRH local double; Rotation local double; LeftRight local double; LXC local double; LYC local double; LZC local double; RXYC local double; safechecker local double; Toggle local double
